simulink model "micro2018b"  (R2018b)
settings: Solver=ode1  StartTime=0.0  StopTime=t_sim  FixedStep=Ts  RelTol=1e-3
values from neighbouring files (symbols this model uses):
  Vo = 200    [param.m]
undefined symbols (not defined in the file or in its folder): C, f_i, fo, L, L1, L2, phi, R, Tm, Ts, Vac_pk
libraries: powerlib x16, powerlib_meascontrol x2, simulink x1, hdlsllib x1
(part 2 of 2)

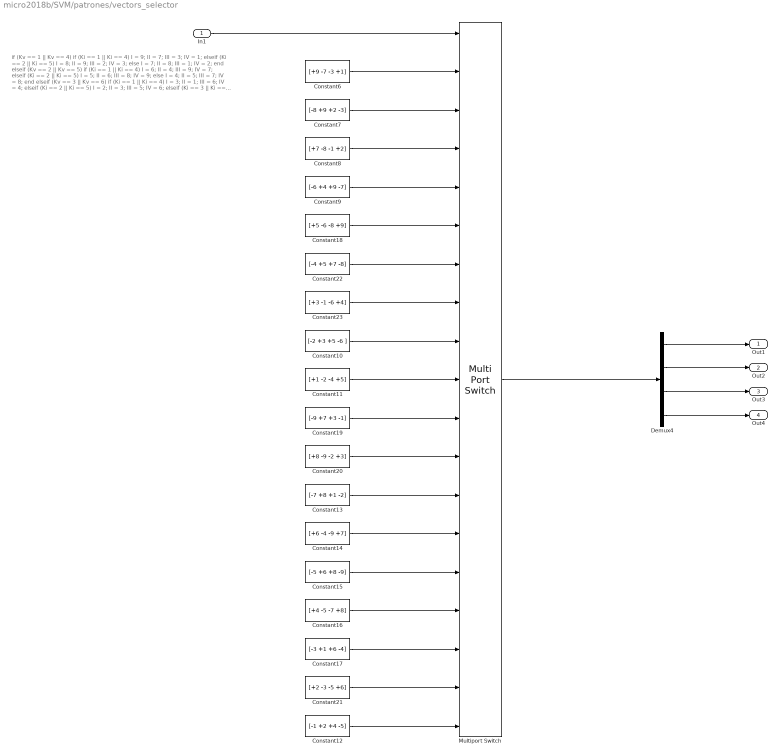
== system micro2018b/SVM/patrones/vectors_selector ==
  note: if (Kv == 1 || Kv == 4)
      | if (Ki == 1 || Ki == 4)
      | I = 9;
      | II = 7;
      | III = 3;
      | IV = 1;
      | elseif (Ki == 2 || Ki == 5)
      | I = 8;
      | II = 9;
      | III = 2;
      | IV = 3;
      | else
      | I = 7;
      | II = 8;
      | III = 1;
      | IV = 2;
      | end
      | elseif (Kv == 2 || Kv == 5)
      | if (Ki == 1 || Ki == 4)
      | I = 6;
      | II = 4;
      | III = 9;
      | IV = 7;
      | elseif (Ki == 2 || Ki == 5)
      | I = 5;
      | II = 6;
      | III = 8;
      | IV = 9;
      | else
      | I = 4;
      | II = 5;
      | III = 7;
      | IV = 8;
      | end
      | elseif (Kv == 3 || Kv == 6)
      | if (Ki == 1 || Ki == 4)
      | I = 3;
      | II = 1;
      | III = 6;
      | IV = 4;
      | elseif (Ki == 2 || Ki == 5)
      | I = 2;
      | II = 3;
      | III = 5;
      | IV = 6;
      | elseif (Ki == 3 || Ki == 6)
      | I = 1;
      | II = 2;
      | III = 4;
      | IV = 5;
      | end
      | end
  In1 : Inport
  Constant10 : Constant  Value=[-2 +3 +5 -6 ]  VectorParams1D=off
  Constant11 : Constant  Value=[+1 -2 -4 +5]  VectorParams1D=off
  Constant12 : Constant  Value=[-1 +2 +4 -5]
  Constant13 : Constant  Value=[-7 +8 +1 -2]
  Constant14 : Constant  Value=[+6 -4 -9 +7]
  Constant15 : Constant  Value=[-5 +6 +8 -9]
  Constant16 : Constant  Value=[+4 -5 -7 +8]  VectorParams1D=off
  Constant17 : Constant  Value=[-3 +1 +6 -4]  VectorParams1D=off
  Constant18 : Constant  Value=[+5 -6 -8 +9]
  Constant19 : Constant  Value=[-9 +7 +3 -1]
  Constant20 : Constant  Value=[+8 -9 -2 +3]
  Constant21 : Constant  Value=[+2 -3 -5 +6]
  Constant22 : Constant  Value=[-4 +5 +7 -8]
  Constant23 : Constant  Value=[+3 -1 -6 +4]  VectorParams1D=off
  Constant6 : Constant  Value=[+9 -7 -3 +1]  VectorParams1D=off
  Constant7 : Constant  Value=[-8 +9 +2 -3]
  Constant8 : Constant  Value=[+7 -8 -1 +2]
  Constant9 : Constant  Value=[-6 +4 +9 -7]
  Demux4 : Demux
  Multiport Switch : MultiPortSwitch  Inputs=18
  Out1 : Outport
  Out2 : Outport  Port=2
  Out3 : Outport  Port=3
  Out4 : Outport  Port=4
  wires:
  Constant15/1 -> Multiport Switch/15
  Multiport Switch/1 -> Demux4/1
  Demux4/2 -> Out2/1
  Constant14/1 -> Multiport Switch/14
  Constant7/1 -> Multiport Switch/3
  Constant9/1 -> Multiport Switch/5
  Constant20/1 -> Multiport Switch/12
  Constant13/1 -> Multiport Switch/13
  Constant10/1 -> Multiport Switch/9
  Constant17/1 -> Multiport Switch/17
  Demux4/1 -> Out1/1
  Constant21/1 -> Multiport Switch/18
  Constant8/1 -> Multiport Switch/4
  Constant16/1 -> Multiport Switch/16
  Constant19/1 -> Multiport Switch/11
  Constant18/1 -> Multiport Switch/6
  Constant6/1 -> Multiport Switch/2
  Constant23/1 -> Multiport Switch/8
  In1/1 -> Multiport Switch/1
  Constant22/1 -> Multiport Switch/7
  Constant11/1 -> Multiport Switch/10
  Constant12/1 -> Multiport Switch/19
  Demux4/4 -> Out4/1
  Demux4/3 -> Out3/1

== system micro2018b/SVM/patrones/vectors_selector1 ==
  note: if (Kv == 1 || Kv == 4)
      | if (Ki == 1 || Ki == 4)
      | I = 9;
      | II = 7;
      | III = 3;
      | IV = 1;
      | elseif (Ki == 2 || Ki == 5)
      | I = 8;
      | II = 9;
      | III = 2;
      | IV = 3;
      | else
      | I = 7;
      | II = 8;
      | III = 1;
      | IV = 2;
      | end
      | elseif (Kv == 2 || Kv == 5)
      | if (Ki == 1 || Ki == 4)
      | I = 6;
      | II = 4;
      | III = 9;
      | IV = 7;
      | elseif (Ki == 2 || Ki == 5)
      | I = 5;
      | II = 6;
      | III = 8;
      | IV = 9;
      | else
      | I = 4;
      | II = 5;
      | III = 7;
      | IV = 8;
      | end
      | elseif (Kv == 3 || Kv == 6)
      | if (Ki == 1 || Ki == 4)
      | I = 3;
      | II = 1;
      | III = 6;
      | IV = 4;
      | elseif (Ki == 2 || Ki == 5)
      | I = 2;
      | II = 3;
      | III = 5;
      | IV = 6;
      | elseif (Ki == 3 || Ki == 6)
      | I = 1;
      | II = 2;
      | III = 4;
      | IV = 5;
      | end
      | end
  In1 : Inport
  Constant10 : Constant  Value=[2 3 5 6 ]  VectorParams1D=off
  Constant11 : Constant  Value=[1 2 4 5]  VectorParams1D=off
  Constant18 : Constant  Value=[5 6 8 9]
  Constant22 : Constant  Value=[4 5 7 8]
  Constant23 : Constant  Value=[3 1 6 4]
  Constant6 : Constant  Value=[9 7 3 1]  VectorParams1D=off
  Constant7 : Constant  Value=[8 9 2 3]
  Constant8 : Constant  Value=[7 8 1 2]
  Constant9 : Constant  Value=[6 4 9 7]
  Demux4 : Demux
  Multiport Switch : MultiPortSwitch  Inputs=9
  Out1 : Outport
  Out2 : Outport  Port=2
  Out3 : Outport  Port=3
  Out4 : Outport  Port=4
  wires:
  Multiport Switch/1 -> Demux4/1
  Demux4/2 -> Out2/1
  Constant7/1 -> Multiport Switch/3
  Constant9/1 -> Multiport Switch/5
  Constant10/1 -> Multiport Switch/9
  Demux4/1 -> Out1/1
  Constant8/1 -> Multiport Switch/4
  Constant18/1 -> Multiport Switch/6
  Constant6/1 -> Multiport Switch/2
  Constant23/1 -> Multiport Switch/8
  In1/1 -> Multiport Switch/1
  Constant22/1 -> Multiport Switch/7
  Constant11/1 -> Multiport Switch/10
  Demux4/4 -> Out4/1
  Demux4/3 -> Out3/1

== matlab function micro2018b/SVM/sectorI ==
  data: Vi_angle input; phi input; angle output; sector output
function [angle, sector] = fcn(Vi_angle, phi)
angle = Vi_angle + phi;
angle = angle + pi/6;
while angle <0
    angle = angle + 2*pi;
end
while angle>2*pi
    angle = angle - 2*pi;
end
sector = 0;
while angle>0
    angle = angle - (pi/3);
    sector = sector + 1;
end
angle = angle + (pi/6);
end

== matlab function micro2018b/SVM/sectorV ==
  data: v_alpha input; angle output; v_beta input; sector output
function [angle, sector] = fcn(v_alpha, v_beta)
    angle = atan2(v_beta, v_alpha);
    if angle<0
        angle = angle + 2*pi;
    end
    sector = 0;
    while (angle>=0)
        angle = angle - (pi/3);
        sector = sector + 1;
    end
    if(sector==7) 
        sector = 1;
    end
    angle = angle + (pi/6);
end

== matlab function micro2018b/SVM/duty_cycle_calculator ==
  data: alpha0 input; Kv input; d1 output; d2 output; d3 output; d4 output; betai input; Ki input; fii input; q input
function [d1, d2, d3, d4] = fcn(alpha0, Kv, betai, Ki, fii, q)
%% calcular los delta
d1 = (-1)^(Kv+Ki)*q*(cos(alpha0 - pi/3)*cos(betai - pi/3)/cos(fii))/1.4;
d2 = (-1)^(Kv+Ki+1) *q*(cos(alpha0 - pi/3)*cos(betai + pi/3)/cos(fii))/1.4;
d3 = (-1)^(Kv+Ki+1) *q*(cos(alpha0 + pi/3)*cos(betai - pi/3)/cos(fii))/1.4;
d4 = (-1)^(Kv+Ki)*q*(cos(alpha0 + pi/3)*cos(betai + pi/3)/cos(fii))/1.4;
end

== matlab function micro2018b/MATLAB Function ==
  data: u input; y output
function y = fcn(u)

x = bitget(u,9:-1:1);

y = x';
